simulink model "VTOLDynamics"  (R2026a)
settings: Solver=VariableStepAuto  StopTime=10
undefined symbols (not defined in the file): battery, contact, env, F, iniRoll, initPitch, iniYaw, Light, MIL, minPWM, motorPID, percWeightGain, tiltIni, uavParam, vIni, xGround, yGround, zGround
libraries: matrix_library x8, robotcorelib x4, aerolibasang x2, aerolibwind2 x2, aerolibobsolete x1, aerolibadyn x1, fl_lib x1, nesl_utility x1, sharedtransform x1
(part 1 of 2)
settings Model: DataDictionary=VTOLDynamicsData.sldd  Creator=The MathWorks, Inc.  LastModifiedBy=The MathWorks, Inc.
settings ModelReferenceCC: ModelReferenceNumInstancesAllowed=Single
settings GRTTargetCC: SubcomponentCodeInterfacePackaging=Nonreusable function
settings SimscapeCC: SimscapeNominalValues="[{\"value\":\"1\",\"unit\":\"A\"},{\"value\":\"1\",\"unit\":\"bar\"},{\"value\":\"1\",\"unit\":\"cm^2\"},{\"value\":\"1\",\"unit\":\"cm^3/s\"},{\"value\":\"1\",\"unit\":\"kJ/kg\"},{\"value\":\"1\",\"unit\":\"kW\"},{\"value\":\"1\",\"unit\":\"l\"},{\"value\":\"1\",\"unit\":\"N\"},{\"value\":\"1\",\"unit\":\"N*m\"},{\"value\":\"1\",\"unit\":\"V\"}]"  SimscapeLogType=none  SimscapeLogDataHistory=5000.0

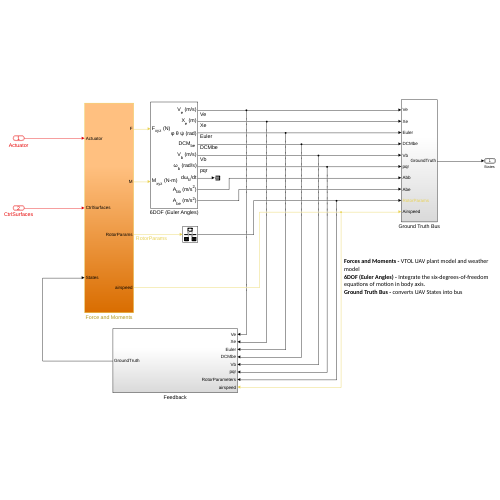
[thumbnail: Simulink's stored preview of the top-level diagram]
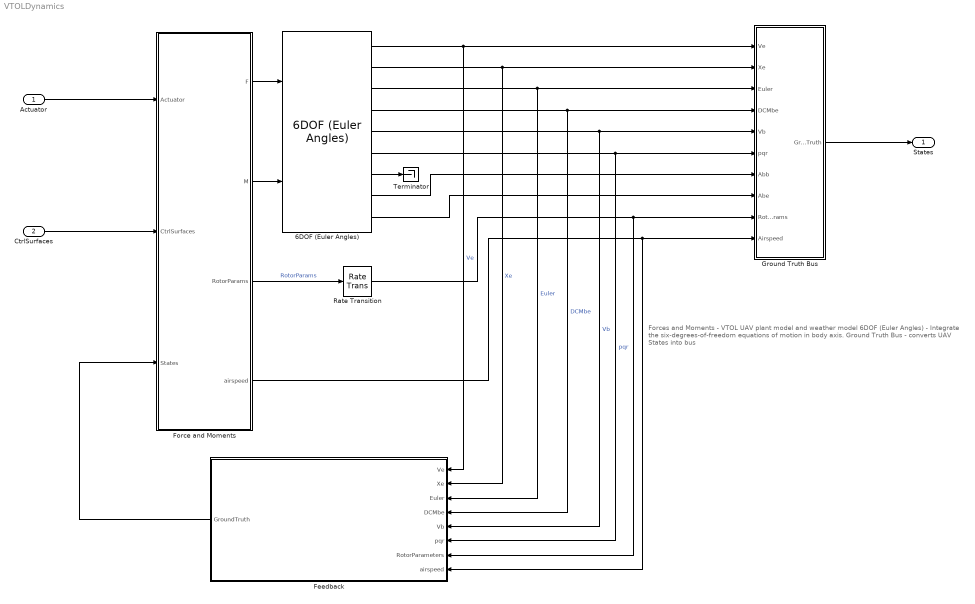
== system VTOLDynamics ==
  note: Forces and Moments - VTOL UAV plant model and weather model
      | 6DOF (Euler Angles) - Integrate the six-degrees-of-freedom equations of motion in body axis.
      | Ground Truth Bus - converts UAV States into bus
  Actuator : Inport  OutDataTypeStr=Bus: RotorCtrlBus  BusOutputAsStruct=on
  CtrlSurfaces : Inport  Port=2  OutDataTypeStr=Bus: FixedWingCtrlBus  BusOutputAsStruct=on
  6DOF (Euler Angles) : aerolibobsolete/6DOF (Euler Angles)  units=Metric (MKS)  mtype=Fixed  rep=Euler Angles  xme_0=[xGround, yGround, zGround]  Vm_0=[vIni 0 0]  eul_0=[iniRoll initPitch iniYaw]  pm_0=[0 0 0]  mass_0=6.031*percWeightGain  mass_e=0.5  mass_f=2.0  inertia=[uavParam.geom.Ixx 0 0; 0 uavParam.geom.Iyy 0; 0 0 uavParam.geom.Izz]  inertia_e=eye(3)  inertia_f=2*eye(3)  k_quat=1.0  vre_flag=on  abi_flag=on  aMode=0  xme_statename=''  Vm_statename=''  eul_statename=''  quat_statename=''  pm_statename=''  mass_statename=''
  Feedback : Subsystem
  Force and Moments : Subsystem
  Ground Truth Bus : Subsystem
  Rate Transition : RateTransition
  Terminator : Terminator
  "States " : Outport  OutDataTypeStr=Bus: stateBus  BusOutputAsStruct=on
  wires:
  6DOF (Euler Angles)/4 -> Feedback/4(DCMbe), Ground Truth Bus/4(DCMbe)  "DCMbe"
  Actuator/1 -> Force and Moments/1(Actuator)
  6DOF (Euler Angles)/2 -> Feedback/2(Xe), Ground Truth Bus/2(Xe)  "Xe"
  Force and Moments/4(airspeed) -> Ground Truth Bus/10(Airspeed), Feedback/8(airspeed)
  6DOF (Euler Angles)/1 -> Feedback/1(Ve), Ground Truth Bus/1(Ve)  "Ve"
  Force and Moments/3(RotorParams) -> Rate Transition/1  "RotorParams"
  6DOF (Euler Angles)/6 -> Feedback/6(pqr), Ground Truth Bus/6(pqr)  "pqr"
  CtrlSurfaces/1 -> Force and Moments/2(CtrlSurfaces)
  6DOF (Euler Angles)/7 -> Terminator/1
  6DOF (Euler Angles)/3 -> Feedback/3(Euler), Ground Truth Bus/3(Euler)  "Euler"
  6DOF (Euler Angles)/5 -> Feedback/5(Vb), Ground Truth Bus/5(Vb)  "Vb"
  Ground Truth Bus/1(GroundTruth) -> "States "/1
  6DOF (Euler Angles)/8 -> Ground Truth Bus/7(Abb)
  6DOF (Euler Angles)/9 -> Ground Truth Bus/8(Abe)
  Feedback/1(GroundTruth) -> Force and Moments/3(States)
  Force and Moments/1(F) -> 6DOF (Euler Angles)/1
  Force and Moments/2(M) -> 6DOF (Euler Angles)/2
  Rate Transition/1 -> Feedback/7(RotorParameters), Ground Truth Bus/9(RotorParams)

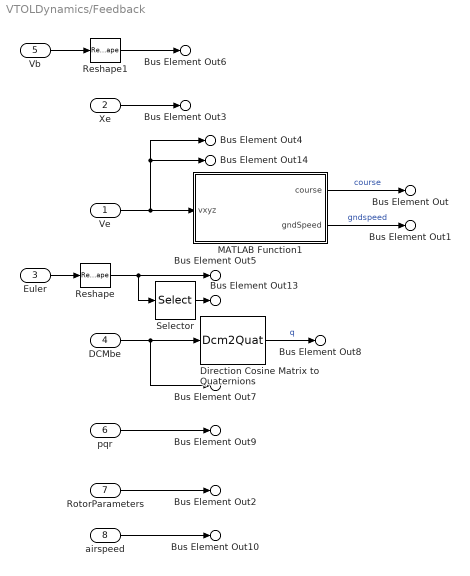
== system VTOLDynamics/Feedback ==
  Ve : Inport
  Xe : Inport  Port=2
  Euler : Inport  Port=3
  DCMbe : Inport  Port=4
  Vb : Inport  Port=5
  pqr : Inport  Port=6
  RotorParameters : Inport  Port=7
  airspeed : Inport  Port=8
  Direction Cosine Matrix to Quaternions : Dcm2Quat
  MATLAB Function1 : MATLAB Function  TreatAsAtomicUnit=on
  Reshape : Reshape  OutputDimensionality=Column vector (2-D)
  Reshape1 : Reshape  OutputDimensionality=Row vector (2-D)
  Selector : Selector  InputPortWidth=3  IndexOptions=Index vector (dialog)  Indices=[3 2 1]  OutputSizes=1
  Bus Element Out : Outport  PortName=GroundTruth  Element=course
  Bus Element Out1 : Outport  PortName=GroundTruth  Element=gndspeed
  Bus Element Out3 : Outport  PortName=GroundTruth  Element=Xe
  Bus Element Out4 : Outport  PortName=GroundTruth  Element=Ve
  Bus Element Out7 : Outport  PortName=GroundTruth  Element=DCMbe
  Bus Element Out8 : Outport  PortName=GroundTruth  Element=q
  Bus Element Out9 : Outport  PortName=GroundTruth  Element=pqr
  Bus Element Out6 : Outport  PortName=GroundTruth  Element=Vb
  Bus Element Out5 : Outport  PortName=GroundTruth  Element=Euler
  Bus Element Out13 : Outport  PortName=GroundTruth  Element=ypr
  Bus Element Out14 : Outport  PortName=GroundTruth  Element=Ve_ground
  Bus Element Out2 : Outport  PortName=GroundTruth  Element=RotorParameters
  Bus Element Out10 : Outport  PortName=GroundTruth  Element=airspeed
  wires:
  Reshape1/1 -> Bus Element Out6/1
  Reshape/1 -> Bus Element Out5/1, Selector/1
  Selector/1 -> Bus Element Out13/1
  pqr/1 -> Bus Element Out9/1
  Direction Cosine Matrix to Quaternions/1 -> Bus Element Out8/1  "q"
  Vb/1 -> Reshape1/1
  Euler/1 -> Reshape/1
  Xe/1 -> Bus Element Out3/1
  MATLAB Function1/2(gndSpeed) -> Bus Element Out1/1  "gndspeed"
  MATLAB Function1/1(course) -> Bus Element Out/1  "course"
  Ve/1 -> MATLAB Function1/1(vxyz), Bus Element Out4/1, Bus Element Out14/1
  DCMbe/1 -> Direction Cosine Matrix to Quaternions/1, Bus Element Out7/1
  RotorParameters/1 -> Bus Element Out2/1
  airspeed/1 -> Bus Element Out10/1

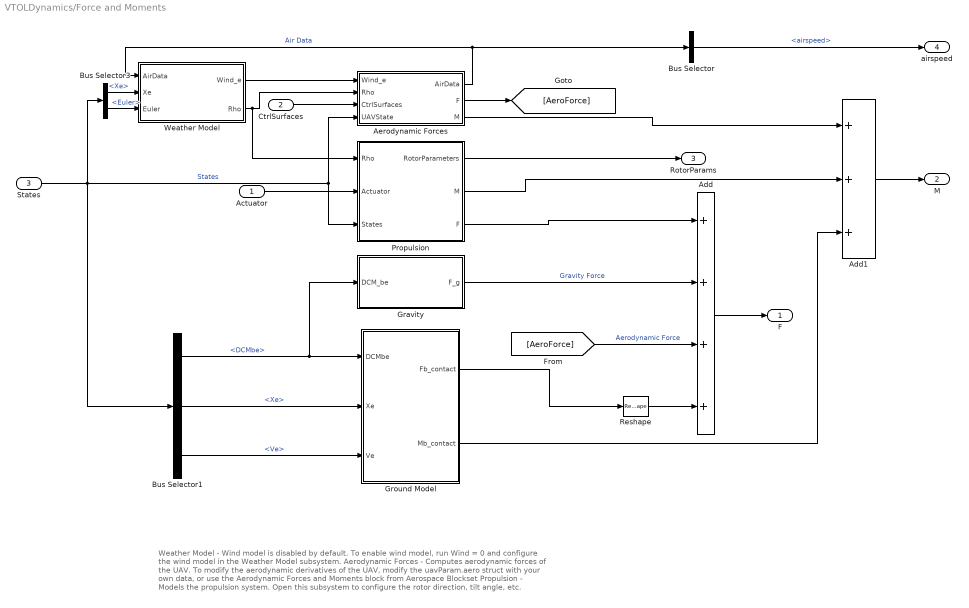
== system VTOLDynamics/Force and Moments ==
  note: Weather Model - Wind model is disabled by default. To enable wind model, run Wind = 0 and configure the wind model in the Weather Model subsystem.
      |
      | Aerodynamic Forces - Computes aerodynamic forces of the UAV. To modify the aerodynamic derivatives of the UAV, modify the uavParam.aero struct with your own data, or use the Aerodynamic Forces and Moments block from Aerospace Blockset
      |
      | Propulsion - Models the propulsion system. Open this subsystem to configure the rotor direction, tilt angle, etc.
  Actuator : Inport
  CtrlSurfaces : Inport  Port=2
  States : Inport  Port=3
  Add : Sum  Inputs=++++
  Add1 : Sum  Inputs=+++
  Aerodynamic Forces : Subsystem
  Bus Selector : BusSelector  OutputSignals=airspeed
  Bus Selector1 : BusSelector  OutputSignals=DCMbe,Xe,Ve
  Bus Selector3 : BusSelector  OutputSignals=Xe,Euler
  Gravity : Subsystem
  Ground Model : Subsystem  VariantControl=Groundon==1
  Propulsion : Subsystem  Variant=on
  Reshape : Reshape
  Weather Model : Subsystem  Variant=on  VariantControl=Weather Model
  F : Outport
  M : Outport  Port=2
  RotorParams : Outport  Port=3
  airspeed : Outport  Port=4
  wires:
  Gravity/1(F_g) -> Add/2  "Gravity Force"
  Add/1 -> F/1
  States/1 -> Bus Selector3/1, Bus Selector1/1, Propulsion/3(States), Aerodynamic Forces/4(UAVState)  "States"
  CtrlSurfaces/1 -> Aerodynamic Forces/3(CtrlSurfaces)
  Add1/1 -> M/1
  [AeroForce] -> Add/3  "Aerodynamic Force"
  Aerodynamic Forces/2(F) -> [AeroForce]
  Aerodynamic Forces/3(M) -> Add1/1
  Aerodynamic Forces/1(AirData) -> Weather Model/1(AirData), Bus Selector/1  "Air Data"
  Bus Selector3/1 -> Weather Model/2(Xe)  "<Xe>"
  Bus Selector3/2 -> Weather Model/3(Euler)  "<Euler>"
  Weather Model/1(Wind_e) -> Aerodynamic Forces/1(Wind_e)
  Weather Model/2(Rho) -> Aerodynamic Forces/2(Rho), Propulsion/1(Rho)
  Bus Selector1/3 -> Ground Model/3(Ve)  "<Ve>"
  Bus Selector1/2 -> Ground Model/2(Xe)  "<Xe>"
  Bus Selector1/1 -> Gravity/1(DCM_be), Ground Model/1(DCMbe)  "<DCMbe>"
  Ground Model/1(Fb_contact) -> Reshape/1
  Ground Model/2(Mb_contact) -> Add1/3
  Reshape/1 -> Add/4
  Bus Selector/1 -> airspeed/1  "<airspeed>"
  Actuator/1 -> Propulsion/2(Actuator)
  Propulsion/2(M) -> Add1/2
  Propulsion/3(F) -> Add/1
  Propulsion/1(RotorParameters) -> RotorParams/1

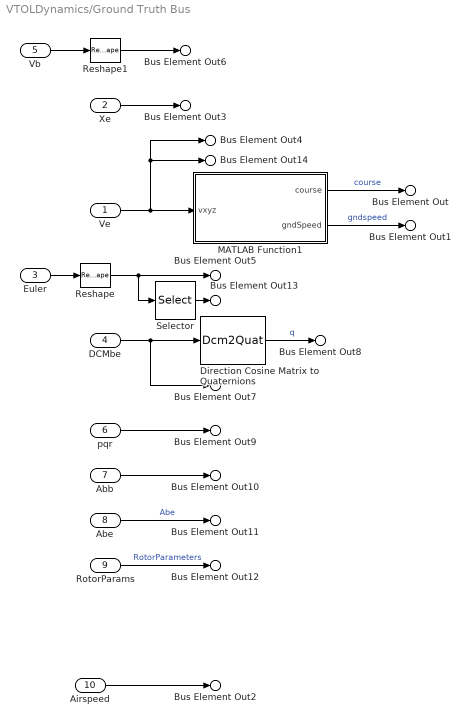
== system VTOLDynamics/Ground Truth Bus ==
  Ve : Inport
  Xe : Inport  Port=2
  Euler : Inport  Port=3
  DCMbe : Inport  Port=4
  Vb : Inport  Port=5
  pqr : Inport  Port=6
  Abb : Inport  Port=7
  Abe : Inport  Port=8
  RotorParams : Inport  Port=9
  Airspeed : Inport  Port=10
  Direction Cosine Matrix to Quaternions : Dcm2Quat
  MATLAB Function1 : MATLAB Function  TreatAsAtomicUnit=on
  Reshape : Reshape  OutputDimensionality=Column vector (2-D)
  Reshape1 : Reshape  OutputDimensionality=Row vector (2-D)
  Selector : Selector  InputPortWidth=3  IndexOptions=Index vector (dialog)  Indices=[3 2 1]  OutputSizes=1
  Bus Element Out : Outport  PortName=GroundTruth  Element=course
  Bus Element Out1 : Outport  PortName=GroundTruth  Element=gndspeed
  Bus Element Out2 : Outport  PortName=GroundTruth  Element=airspeed
  Bus Element Out3 : Outport  PortName=GroundTruth  Element=Xe
  Bus Element Out4 : Outport  PortName=GroundTruth  Element=Ve
  Bus Element Out7 : Outport  PortName=GroundTruth  Element=DCMbe
  Bus Element Out8 : Outport  PortName=GroundTruth  Element=q
  Bus Element Out9 : Outport  PortName=GroundTruth  Element=pqr
  Bus Element Out6 : Outport  PortName=GroundTruth  Element=Vb
  Bus Element Out10 : Outport  PortName=GroundTruth  Element=Abb
  Bus Element Out11 : Outport  PortName=GroundTruth  Element=Abe
  Bus Element Out5 : Outport  PortName=GroundTruth  Element=Euler
  Bus Element Out12 : Outport  PortName=GroundTruth  Element=RotorParameters
  Bus Element Out13 : Outport  PortName=GroundTruth  Element=ypr
  Bus Element Out14 : Outport  PortName=GroundTruth  Element=Ve_ground
  wires:
  DCMbe/1 -> Bus Element Out7/1, Direction Cosine Matrix to Quaternions/1
  Airspeed/1 -> Bus Element Out2/1
  Ve/1 -> Bus Element Out14/1, Bus Element Out4/1, MATLAB Function1/1(vxyz)
  MATLAB Function1/1(course) -> Bus Element Out/1  "course"
  MATLAB Function1/2(gndSpeed) -> Bus Element Out1/1  "gndspeed"
  Xe/1 -> Bus Element Out3/1
  Euler/1 -> Reshape/1
  Vb/1 -> Reshape1/1
  Direction Cosine Matrix to Quaternions/1 -> Bus Element Out8/1  "q"
  pqr/1 -> Bus Element Out9/1
  Abb/1 -> Bus Element Out10/1
  Abe/1 -> Bus Element Out11/1  "Abe"
  RotorParams/1 -> Bus Element Out12/1  "RotorParameters"
  Selector/1 -> Bus Element Out13/1
  Reshape/1 -> Selector/1, Bus Element Out5/1
  Reshape1/1 -> Bus Element Out6/1

== system VTOLDynamics/Force and Moments/Aerodynamic Forces ==
  Wind_e : Inport
  Rho : Inport  Port=2
  CtrlSurfaces : Inport  Port=3
  UAVState : Inport  Port=4
  Bus Selector2 : BusSelector  OutputSignals=DCMbe,Ve,pqr
  Compute Air Data : Subsystem  TreatAsAtomicUnit=on  VariantControl=use_aerospace_blocks == 1
  Compute Body Frame Forces and Moments : Subsystem
  Matrix Multiply : Product  Multiplication=Matrix(*)
  Vair : Sum  Inputs=+-  InputSameDT=on  SaturateOnIntegerOverflow=on  OutDataTypeStr=Inherit: Same as first input
  AirData : Outport  VectorParamsAs1DForOutWhenUnconnected=off
  F : Outport  Port=2
  M : Outport  Port=3
  wires:
  Bus Selector2/2 -> Vair/1  "<Ve>"
  UAVState/1 -> Bus Selector2/1
  Compute Body Frame Forces and Moments/1(F_b) -> F/1
  CtrlSurfaces/1 -> Compute Body Frame Forces and Moments/2(CtrlSurfaces)
  Compute Air Data/1(AirData) -> Compute Body Frame Forces and Moments/1(AirData), AirData/1
  Bus Selector2/3 -> Compute Body Frame Forces and Moments/4(p,q,r)  "<pqr>"
  Compute Body Frame Forces and Moments/2(M_b) -> M/1
  Matrix Multiply/1 -> Compute Body Frame Forces and Moments/3(Vb), Compute Air Data/1(Vb)
  Rho/1 -> Compute Air Data/2(Rho)
  Vair/1 -> Matrix Multiply/2
  Bus Selector2/1 -> Matrix Multiply/1  "<DCMbe>"
  Wind_e/1 -> Vair/2

== system VTOLDynamics/Force and Moments/Gravity ==
  DCM_be : Inport
  Constant : Constant  Value=[0 0 uavParam.aero.g]'
  Gain : Gain  Gain=uavParam.geom.mass*percWeightGain
  Matrix Multiply : Product  Multiplication=Matrix(*)
  F_g : Outport
  wires:
  Matrix Multiply/1 -> Gain/1
  Constant/1 -> Matrix Multiply/2
  DCM_be/1 -> Matrix Multiply/1
  Gain/1 -> F_g/1

== system VTOLDynamics/Force and Moments/Ground Model ==
  note: Body is assumed to be a rigid point mass on ground for contact force calculations.
      |
      | Normal force is modelled as a spring mass damper.
      |
      | Friction is modelled using Soft Coulomb model.
  DCMbe : Inport
  Xe : Inport  Port=2
  Ve : Inport  Port=3
  Constant : Constant  Value=[0 0 0]  SampleTime=-1
  Friction Force : Subsystem
  Matrix Multiply : Product  Multiplication=Matrix(*)
  Mux1 : Mux  Inputs=2
  Normal Force : Subsystem
  Selector : Selector  InputPortWidth=3  IndexOptions=Index vector (dialog)  Indices=[3]  OutputSizes=1
  Selector1 : Selector  InputPortWidth=3  IndexOptions=Index vector (dialog)  Indices=[3]  OutputSizes=1
  Selector2 : Selector  InputPortWidth=3  IndexOptions=Index vector (dialog)  Indices=[1,2]  OutputSizes=1
  Unary Minus1 : UnaryMinus
  Fb_contact : Outport
  Mb_contact : Outport  Port=2
  wires:
  Xe/1 -> Selector/1
  Ve/1 -> Selector2/1, Selector1/1
  Selector1/1 -> Normal Force/1(Vz)
  Selector/1 -> Normal Force/2(Z)
  DCMbe/1 -> Matrix Multiply/1
  Matrix Multiply/1 -> Fb_contact/1
  Normal Force/1(Normal) -> Friction Force/2(Fn), Unary Minus1/1
  Mux1/1 -> Matrix Multiply/2
  Unary Minus1/1 -> Mux1/2
  Selector2/1 -> Friction Force/1(V)
  Friction Force/1(Friction) -> Mux1/1
  Constant/1 -> Mb_contact/1

== system VTOLDynamics/Force and Moments/Propulsion ==
  note: 1) Add Subsystem or Model blocks as valid variant choices.
      | 2) You cannot connect blocks at this level. At simulation, connectivity is automatically
      | determined, based on the active variant and port name matching.
  Rho : Inport
  Actuator : Inport  Port=2
  States : Inport  Port=3
  Electric Propulsion : Subsystem  VariantControl=ElectricPropulsion == 1
  Propulsion : Subsystem  VariantControl=ElectricPropulsion == 0
  RotorParameters : Outport
  M : Outport  Port=2
  F : Outport  Port=3

== system VTOLDynamics/Force and Moments/Weather Model ==
  AirData : Inport
  Xe : Inport  Port=2
  Euler : Inport  Port=3
  Simple Model : Subsystem  VariantControl=Wind==0
  Weather Model : Subsystem  VariantControl=Wind==1
  Wind_e : Outport
  Rho : Outport  Port=2

== system VTOLDynamics/Force and Moments/Aerodynamic Forces/Compute Air Data ==
  Vb : Inport  PortDimensions=3
  Rho : Inport  Port=2
  Bus Creator : BusCreator  Inputs=4
  Constant : Constant  Value=5/57.296
  Dynamic Pressure : aerolibasang/Dynamic Pressure
  "Incidence, Sideslip, & Airspeed" : aerolibasang/Incidence, Sideslip, & Airspeed
  Saturation : Saturate  UpperLimit=14*pi/180  LowerLimit=-14*pi/180
  Sum : Sum  Inputs=|++
  To Workspace : ToWorkspace  VariableName=Alpha  SaveFormat=Timeseries  SampleTime=-1
  AirData : Outport  VectorParamsAs1DForOutWhenUnconnected=off
  wires:
  Bus Creator/1 -> AirData/1
  "Incidence, Sideslip, & Airspeed"/1 -> Sum/2, Bus Creator/1  "alpha"
  Rho/1 -> Dynamic Pressure/2
  "Incidence, Sideslip, & Airspeed"/3 -> Bus Creator/3  "airspeed"
  Dynamic Pressure/1 -> Bus Creator/4  "q"
  Vb/1 -> "Incidence, Sideslip, & Airspeed"/1, Dynamic Pressure/1
  "Incidence, Sideslip, & Airspeed"/2 -> Saturation/1  "beta"
  Saturation/1 -> Bus Creator/2  "beta"
  Constant/1 -> Sum/1
  Sum/1 -> To Workspace/1

== system VTOLDynamics/Force and Moments/Aerodynamic Forces/Compute Body Frame Forces and Moments ==
  AirData : Inport
  CtrlSurfaces : Inport  Port=2
  Vb : Inport  Port=3
  p,q,r : Inport  Port=4
  "Aerodynamic Forces and Moments " : aerolibadyn/Aerodynamic Forces and Moments   inputAxes=Wind  outputForceAxes=Body  outputMomentAxes=Body  S=uavParam.geom.b*uavParam.geom.c  b=uavParam.geom.b  cbar=uavParam.geom.c
  Constant1 : Constant  Value=[0 0 0]
  Constant2 : Constant  Value=[0 0 0]
  Wind frame F& M : Subsystem
  F_b : Outport  Unit=kg*m/s^2  VectorParamsAs1DForOutWhenUnconnected=off
  M_b : Outport  Port=2  Unit=kg*m/s  VectorParamsAs1DForOutWhenUnconnected=off
  wires:
  p,q,r/1 -> Wind frame F& M/3(p,q,r)
  "Aerodynamic Forces and Moments "/2 -> M_b/1
  "Aerodynamic Forces and Moments "/1 -> F_b/1
  CtrlSurfaces/1 -> Wind frame F& M/2(CtrlSurfaces)
  AirData/1 -> Wind frame F& M/1(Airdata)
  Vb/1 -> "Aerodynamic Forces and Moments "/5
  Constant1/1 -> "Aerodynamic Forces and Moments "/3
  Constant2/1 -> "Aerodynamic Forces and Moments "/4
  Wind frame F& M/1(coef) -> "Aerodynamic Forces and Moments "/1  "FM_W"
  Wind frame F& M/2(q) -> "Aerodynamic Forces and Moments "/2

== system VTOLDynamics/Force and Moments/Ground Model/Friction Force ==
  V : Inport
  Fn : Inport  Port=2
  Product : Product
  Soft Coulomb Friction : Subsystem
  Unary Minus : UnaryMinus
  Friction : Outport
  wires:
  Unary Minus/1 -> Friction/1
  Fn/1 -> Product/2
  Soft Coulomb Friction/1(Out1) -> Product/1
  Product/1 -> Unary Minus/1
  V/1 -> Soft Coulomb Friction/1(V)

== system VTOLDynamics/Force and Moments/Ground Model/Normal Force ==
  Vz : Inport
  Z : Inport  Port=2
  Add : Sum
  Constant : Constant  Value=0  SampleTime=-1
  Damper : Gain  Gain=-sqrt(contact.spring*uavParam.geom.mass)
  Saturation : Saturate  UpperLimit=inf  LowerLimit=0  ZeroCross=off
  Spring Kp : Gain  Gain=-contact.spring
  Switch : Switch  Criteria=u2 > Threshold  SaturateOnIntegerOverflow=off  InputSameDT=off
  Unary Minus : UnaryMinus
  Unary Minus1 : UnaryMinus
  Normal : Outport
  wires:
  Add/1 -> Switch/3
  Constant/1 -> Switch/1
  Z/1 -> Unary Minus/1
  Switch/1 -> Saturation/1
  Damper/1 -> Add/2
  Spring Kp/1 -> Add/1
  Vz/1 -> Unary Minus1/1
  Saturation/1 -> Normal/1
  Unary Minus/1 -> Spring Kp/1, Switch/2
  Unary Minus1/1 -> Damper/1

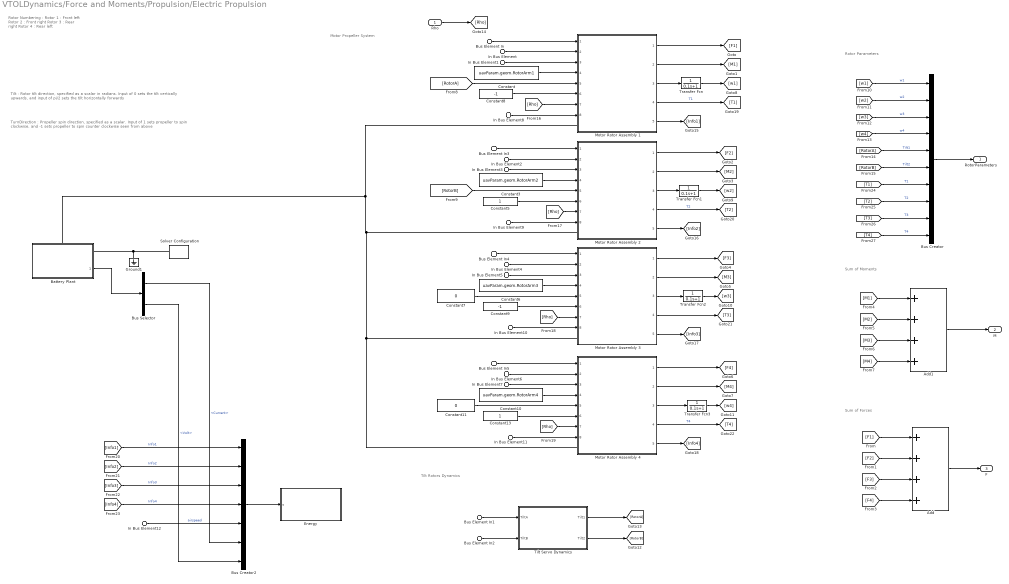
== system VTOLDynamics/Force and Moments/Propulsion/Electric Propulsion ==
  note: Rotor Parameters
  note: Sum of Forces
  note: Sum of Moments
  note: Tilt Rotors Dynamics
  note: Rotor Numbering :
      | Rotor 1 : Front left
      | Rotor 2 : Front right
      | Rotor 3 : Rear right
      | Rotor 4 : Rear left
  note: Tilt : Rotor tilt direction, specified as a scalar in radians. Input of 0 sets the tilt vertically upwards, and input of pi/2 sets the tilt horizontally forwards
  note: TurnDirection : Propeller spin direction, specified as a scalar. Input of 1 sets propeller to spin clockwise, and -1 sets propeller to spin counter clockwise seen from above
  note: Motor Propeller
      | System
  Rho : Inport
  Bus Element In : Inport  Port=2  PortName=Actuator  Element=w1
  Bus Element In1 : Inport  Port=2  PortName=Actuator  Element=Tilt1
  Bus Element In2 : Inport  Port=2  PortName=Actuator  Element=Tilt2
  Bus Element In3 : Inport  Port=2  PortName=Actuator  Element=w2
  Bus Element In5 : Inport  Port=2  PortName=Actuator  Element=w4
  Bus Element In4 : Inport  Port=2  PortName=Actuator  Element=w3
  In Bus Element{,2,4,6} (4 alike) : Inport  Port=3  PortName=States  Element=Vb
  In Bus Element{1,3,5,7} (4 alike) : Inport  Port=3  PortName=States  Element=pqr
  In Bus Element8 : Inport  Port=3  PortName=States  Element=RotorParameters.T1
  In Bus Element9 : Inport  Port=3  PortName=States  Element=RotorParameters.T2
  In Bus Element10 : Inport  Port=3  PortName=States  Element=RotorParameters.T3
  In Bus Element11 : Inport  Port=3  PortName=States  Element=RotorParameters.T4
  In Bus Element12 : Inport  Port=3  PortName=States  Element=airspeed
  Add : Sum  Inputs=++++
  Add1 : Sum  Inputs=++++
  Battery Plant : Subsystem  ReferencedSubsystem=BatteryPlantModel_Simple
      settings: PortSchema="{\"entries\":[{\"content\":{\"sides\":[{\"content\":{},\"type\":\"ConnectorPlacement.EquallySpacedRectSide\",\"uuid\":\"ba36f307-b33b-4535-ba0b-2e0bfd99fc4d\"},{\"content\":{\"connectorIds\":[\"RConn2\",\"Out1\"],\"side\":\"RIGHT\"},\"type\":\"ConnectorPlacement.EquallySpacedRectSide\",\"uuid\":\"89704593-04c2-4c1a-a3b9-13b3f56a74b5\"},{\"content\":{\"connectorIds\":[\"RConn1\"],\"side\":\"TOP\"},\"type\":\"ConnectorPlacement.EquallySpacedRectSide\",\"uuid\":\"1daeac74-7d2b-4aa4-8837-06dc1649b516\"},{\"content\":{\"side\":\"BOTTOM\"},\"type\":\"ConnectorPlacement.EquallySpacedRectSide\",\"uuid\":\"a55355a8-f534-49c8-a897-d3f7ff506222\"}]},\"type\":\"ConnectorPlacement.EquallySpacedConnector\",\"uuid\":\"2c693ef8-3b08-48d7-935c-b55223a280fc\"}],\"packageUris\":[\"http://schema.mathworks.com/mf0/Connector/R2020b\"],\"version\":\"1.0\"}"
  Bus Creator : BusCreator  Inputs=10  OutDataTypeStr=Bus: RotorCtrlBus
  Bus Creator2 : BusCreator  Inputs=7
  Bus Selector : BusSelector  OutputSignals=Current,Volt
  Constant : Constant  Value=uavParam.geom.RotorArm1
  Constant10 : Constant  Value=uavParam.geom.RotorArm4
  Constant11 : Constant  Value=0
  Constant13 : Constant
  Constant3 : Constant  Value=uavParam.geom.RotorArm2
  Constant5 : Constant
  Constant6 : Constant  Value=uavParam.geom.RotorArm3
  Constant7 : Constant  Value=0
  Constant8 : Constant  Value=-1
  Constant9 : Constant  Value=-1
  Energy : Subsystem
      mask Display:
      | %disp(get_param(gcb, 'Name'))
      | disp(['{\bf\fontsize{12}' get_param(gcb, 'Name') '}'], 'texmode','on');
  Ground1 : fl_lib/Electrical/Electrical Elements/Electrical Reference
  Motor Rotor Assembly {1..4} (4 alike) : Subsystem  ReferencedSubsystem=MotorPropellerSystem  Kp=motorPID.Kpp  Ki=motorPID.Kii  Kd=motorPID.Kdd  N=motorPID.N
  Solver Configuration : nesl_utility/Solver Configuration  PhysicalDomain=network_engine_domain  SubClassName=solver  LeftPortType=input  RightPortType=generic  Tones=[]  Harmonics=[]  SimulateNoise=off  Profile=off  UseLocalSampling=off  EnableSwitchedLinearOptims=on  FrequencyDomain=off  UseCCode=off  RelTol=0.001  AbsTol=0.001  MinStep=1e-09  ToWorkspace=off  RevertToSquareIcSolve=off  NumHomotopyIterations=100  PhasorMode=off  PhasorModeNumHarmonics=1  ConsistencySolver=NEWTON_XTOL_AFTER_FTOL  CanonicalOrdering=UNORDERED  OptimizeIntermediates=UNOPTIMIZED  IndexReductionMethod=DerivativeReplacement  DoDC=off  ResidualTolerance=1e-09  ConsistencyTolSource=GLOBAL  ConsistencyAbsTol=0.001  ConsistencyRelTol=0.001  ConsistencyTolFactor=0.001  UseLocalSolver=on  LocalSolverChoice=NE_BACKWARD_EULER_ADVANCER  ResolveIndetEquations=on  FunctionEvalNumThread=1  LocalSolverSampleTime=0.01  DoFixedCost=off  MaxNonlinIter=3  MaxModeIter=2  ComputeImpulses=off  ImpulseIterations=2  LinearAlgebra=auto  LinearAlgebraNumThread=0  EquationFormulation=NE_TIME_EF  DelaysMemoryBudget=1024  AutomaticFiltering=on  FilteringTimeConstant=0.001  PartitionStorageMethod=AS_NEEDED  PartitionMemoryBudget=1024  PartitionMethod=ROBUST  MultibodyUseLocalSolver=off  MultibodyLocalSolverChoice=ODE1  MultibodyLocalSolverSampleTime=0.001
  Tilt Servo Dynamics : Subsystem
  Transfer Fcn{,1..3} (4 alike) : TransferFcn  Denominator=[0.1 1]
  RotorParameters : Outport
  M : Outport  Port=2
  F : Outport  Port=3
  wires:
  [Rho] -> Motor Rotor Assembly 4/7
  [Rho] -> Motor Rotor Assembly 2/7
  [RotorB] -> Motor Rotor Assembly 2/5
  [Rho] -> Motor Rotor Assembly 1/7
  Rho/1 -> [Rho]
  Transfer Fcn3/1 -> [w4]
  Transfer Fcn2/1 -> [w3]
  Transfer Fcn1/1 -> [w2]
  Transfer Fcn/1 -> [w1]
  Bus Element In2/1 -> Tilt Servo Dynamics/2(TiltB)
  Bus Element In1/1 -> Tilt Servo Dynamics/1(TiltA)
  Tilt Servo Dynamics/2(Tilt2) -> [RotorB]
  Tilt Servo Dynamics/1(Tilt1) -> [RotorA]
  Bus Element In5/1 -> Motor Rotor Assembly 4/1
  Bus Element In3/1 -> Motor Rotor Assembly 2/1
  Bus Element In/1 -> Motor Rotor Assembly 1/1
  [RotorB] -> Bus Creator/6  "Tilt2"
  [RotorA] -> Bus Creator/5  "Tilt1"
  Bus Creator/1 -> RotorParameters/1
  [w4] -> Bus Creator/4  "w4"
  [w3] -> Bus Creator/3  "w3"
  [w2] -> Bus Creator/2  "w2"
  [w1] -> Bus Creator/1  "w1"
  Motor Rotor Assembly 4/3 -> Transfer Fcn3/1
  Motor Rotor Assembly 2/3 -> Transfer Fcn1/1
  Motor Rotor Assembly 1/3 -> Transfer Fcn/1
  [M1] -> Add1/1
  [M2] -> Add1/2
  [M3] -> Add1/3
  Add1/1 -> M/1
  [M4] -> Add1/4
  [F4] -> Add/4
  [F3] -> Add/3
  [F2] -> Add/2
  [F1] -> Add/1
  Motor Rotor Assembly 4/2 -> [M4]
  In Bus Element7/1 -> Motor Rotor Assembly 4/3
  Constant11/1 -> Motor Rotor Assembly 4/5
  Constant13/1 -> Motor Rotor Assembly 4/6
  Constant10/1 -> Motor Rotor Assembly 4/4
  In Bus Element6/1 -> Motor Rotor Assembly 4/2
  Motor Rotor Assembly 4/1 -> [F4]
  Motor Rotor Assembly 2/2 -> [M2]
  In Bus Element3/1 -> Motor Rotor Assembly 2/3
  Constant5/1 -> Motor Rotor Assembly 2/6
  Constant3/1 -> Motor Rotor Assembly 2/4
  In Bus Element2/1 -> Motor Rotor Assembly 2/2
  Motor Rotor Assembly 2/1 -> [F2]
  Motor Rotor Assembly 1/2 -> [M1]
  Motor Rotor Assembly 1/1 -> [F1]
  Constant8/1 -> Motor Rotor Assembly 1/6
  Add/1 -> F/1
  [RotorA] -> Motor Rotor Assembly 1/5
  Constant/1 -> Motor Rotor Assembly 1/4
  In Bus Element1/1 -> Motor Rotor Assembly 1/3
  In Bus Element/1 -> Motor Rotor Assembly 1/2
  Battery Plant/1 -> Bus Selector/1
  In Bus Element9/1 -> Motor Rotor Assembly 2/8
  In Bus Element8/1 -> Motor Rotor Assembly 1/8
  In Bus Element11/1 -> Motor Rotor Assembly 4/8
  Motor Rotor Assembly 1/5 -> [Info1]
  Motor Rotor Assembly 2/5 -> [Info2]
  Motor Rotor Assembly 4/5 -> [Info4]
  [Info1] -> Bus Creator2/1  "Info1"
  [Info2] -> Bus Creator2/2  "Info2"
  [Info3] -> Bus Creator2/3  "Info3"
  [Info4] -> Bus Creator2/4  "Info4"
  In Bus Element12/1 -> Bus Creator2/5  "airspeed"
  Bus Selector/1 -> Bus Creator2/6  "<Current>"
  Bus Selector/2 -> Bus Creator2/7  "<Volt>"
  Bus Creator2/1 -> Energy/1(s)
  Motor Rotor Assembly 1/4 -> [T1]  "T1"
  Motor Rotor Assembly 2/4 -> [T2]  "T2"
  Motor Rotor Assembly 4/4 -> [T4]  "T4"
  [T1] -> Bus Creator/7  "T1"
  [T2] -> Bus Creator/8  "T2"
  [T3] -> Bus Creator/9  "T3"
  [T4] -> Bus Creator/10  "T4"
  Bus Element In4/1 -> Motor Rotor Assembly 3/1
  In Bus Element4/1 -> Motor Rotor Assembly 3/2
  In Bus Element5/1 -> Motor Rotor Assembly 3/3
  Constant6/1 -> Motor Rotor Assembly 3/4
  Constant7/1 -> Motor Rotor Assembly 3/5
  Constant9/1 -> Motor Rotor Assembly 3/6
  [Rho] -> Motor Rotor Assembly 3/7
  In Bus Element10/1 -> Motor Rotor Assembly 3/8
  Motor Rotor Assembly 3/5 -> [Info3]
  Motor Rotor Assembly 3/4 -> [T3]
  Motor Rotor Assembly 3/3 -> Transfer Fcn2/1
  Motor Rotor Assembly 3/2 -> [M3]
  Motor Rotor Assembly 3/1 -> [F3]
  connections:
  Solver Configuration/RConn1 -- Ground1/LConn1 -- Battery Plant/RConn2
  Motor Rotor Assembly 1/LConn1 -- Battery Plant/RConn1 -- Motor Rotor Assembly 2/LConn1 -- Motor Rotor Assembly 4/LConn1 -- Motor Rotor Assembly 3/LConn1

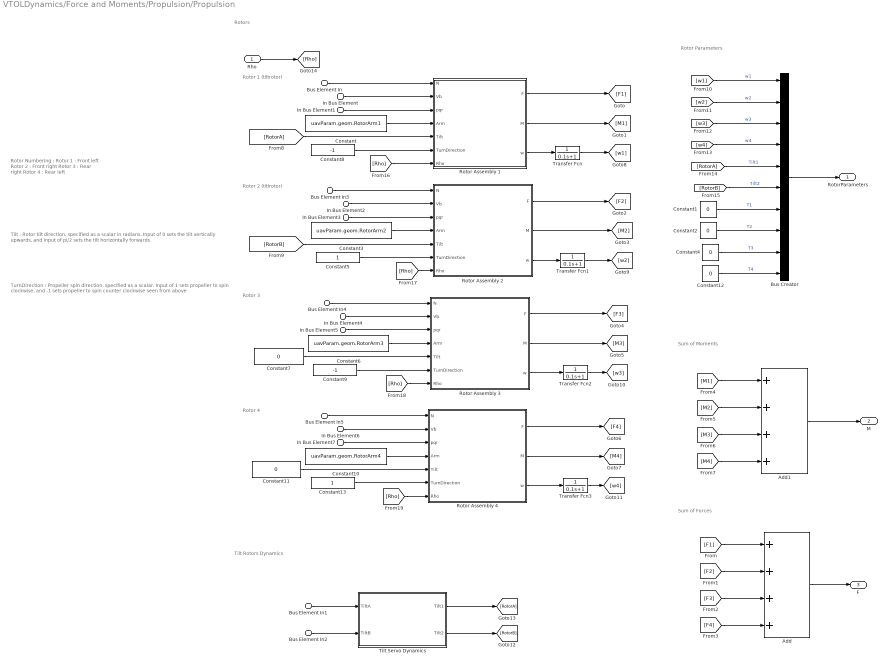
== system VTOLDynamics/Force and Moments/Propulsion/Propulsion ==
  note: TurnDirection : Propeller spin direction, specified as a scalar. Input of 1 sets propeller to spin clockwise, and -1 sets propeller to spin counter clockwise seen from above
  note: Tilt : Rotor tilt direction, specified as a scalar in radians. Input of 0 sets the tilt vertically upwards, and input of pi/2 sets the tilt horizontally forwards
  note: Rotor Numbering :
      | Rotor 1 : Front left
      | Rotor 2 : Front right
      | Rotor 3 : Rear right
      | Rotor 4 : Rear left
  note: Tilt Rotors Dynamics
  note: Sum of Moments
  note: Rotor 1
      | (tiltrotor)
  note: Rotors
  note: Rotor 2
      | (titlrotor)
  note: Rotor 3
  note: Rotor 4
  note: Sum of Forces
  note: Rotor Parameters
  Rho : Inport
  Bus Element In : Inport  Port=2  PortName=Actuator  Element=w1
  Bus Element In1 : Inport  Port=2  PortName=Actuator  Element=Tilt1
  Bus Element In2 : Inport  Port=2  PortName=Actuator  Element=Tilt2
  Bus Element In3 : Inport  Port=2  PortName=Actuator  Element=w2
  Bus Element In5 : Inport  Port=2  PortName=Actuator  Element=w4
  Bus Element In4 : Inport  Port=2  PortName=Actuator  Element=w3
  In Bus Element{,2,4,6} (4 alike) : Inport  Port=3  PortName=States  Element=Vb
  In Bus Element{1,3,5,7} (4 alike) : Inport  Port=3  PortName=States  Element=pqr
  Add : Sum  Inputs=++++
  Add1 : Sum  Inputs=++++
  Bus Creator : BusCreator  Inputs=10  OutDataTypeStr=Bus: RotorCtrlBus
  Constant : Constant  Value=uavParam.geom.RotorArm1
  Constant{1..2,4,7,11..12} (6 alike) : Constant  Value=0
  Constant10 : Constant  Value=uavParam.geom.RotorArm4
  Constant13 : Constant
  Constant3 : Constant  Value=uavParam.geom.RotorArm2
  Constant5 : Constant
  Constant6 : Constant  Value=uavParam.geom.RotorArm3
  Constant8 : Constant  Value=-1
  Constant9 : Constant  Value=-1
  Rotor Assembly 1 : Subsystem
  Rotor Assembly 2 : Subsystem
  "Rotor Assembly 3 " : Subsystem
  Rotor Assembly 4 : Subsystem
  Tilt Servo Dynamics : Subsystem
  Transfer Fcn{,1..3} (4 alike) : TransferFcn  Denominator=[0.1 1]
  RotorParameters : Outport
  M : Outport  Port=2
  F : Outport  Port=3
  wires:
  In Bus Element/1 -> Rotor Assembly 1/2(Vb)
  In Bus Element1/1 -> Rotor Assembly 1/3(pqr)
  Constant/1 -> Rotor Assembly 1/4(Arm)
  [RotorA] -> Rotor Assembly 1/5(Tilt)
  Add/1 -> F/1
  Constant8/1 -> Rotor Assembly 1/6(TurnDirection)
  Rotor Assembly 1/1(F) -> [F1]
  Rotor Assembly 1/2(M) -> [M1]
  Rotor Assembly 2/1(F) -> [F2]
  In Bus Element2/1 -> Rotor Assembly 2/2(Vb)
  Constant3/1 -> Rotor Assembly 2/4(Arm)
  Constant5/1 -> Rotor Assembly 2/6(TurnDirection)
  In Bus Element3/1 -> Rotor Assembly 2/3(pqr)
  Rotor Assembly 2/2(M) -> [M2]
  "Rotor Assembly 3 "/1(F) -> [F3]
  In Bus Element4/1 -> "Rotor Assembly 3 "/2(Vb)
  Constant6/1 -> "Rotor Assembly 3 "/4(Arm)
  Constant9/1 -> "Rotor Assembly 3 "/6(TurnDirection)
  Constant7/1 -> "Rotor Assembly 3 "/5(Tilt)
  In Bus Element5/1 -> "Rotor Assembly 3 "/3(pqr)
  "Rotor Assembly 3 "/2(M) -> [M3]
  Rotor Assembly 4/1(F) -> [F4]
  In Bus Element6/1 -> Rotor Assembly 4/2(Vb)
  Constant10/1 -> Rotor Assembly 4/4(Arm)
  Constant13/1 -> Rotor Assembly 4/6(TurnDirection)
  Constant11/1 -> Rotor Assembly 4/5(Tilt)
  In Bus Element7/1 -> Rotor Assembly 4/3(pqr)
  Rotor Assembly 4/2(M) -> [M4]
  [F1] -> Add/1
  [F2] -> Add/2
  [F3] -> Add/3
  [F4] -> Add/4
  [M4] -> Add1/4
  Add1/1 -> M/1
  [M3] -> Add1/3
  [M2] -> Add1/2
  [M1] -> Add1/1
  Rotor Assembly 1/3(w) -> Transfer Fcn/1
  Rotor Assembly 2/3(w) -> Transfer Fcn1/1
  "Rotor Assembly 3 "/3(w) -> Transfer Fcn2/1
  Rotor Assembly 4/3(w) -> Transfer Fcn3/1
  Bus Element In/1 -> Rotor Assembly 1/1(N)
  Bus Element In3/1 -> Rotor Assembly 2/1(N)
  Bus Element In4/1 -> "Rotor Assembly 3 "/1(N)
  Bus Element In5/1 -> Rotor Assembly 4/1(N)
  Tilt Servo Dynamics/1(Tilt1) -> [RotorA]
  Tilt Servo Dynamics/2(Tilt2) -> [RotorB]
  Bus Element In1/1 -> Tilt Servo Dynamics/1(TiltA)
  Bus Element In2/1 -> Tilt Servo Dynamics/2(TiltB)
  Transfer Fcn/1 -> [w1]
  Transfer Fcn1/1 -> [w2]
  Transfer Fcn2/1 -> [w3]
  Transfer Fcn3/1 -> [w4]
  Rho/1 -> [Rho]
  [Rho] -> Rotor Assembly 1/7(Rho)
  [RotorB] -> Rotor Assembly 2/5(Tilt)
  [Rho] -> Rotor Assembly 2/7(Rho)
  [Rho] -> "Rotor Assembly 3 "/7(Rho)
  [Rho] -> Rotor Assembly 4/7(Rho)
  [w1] -> Bus Creator/1  "w1"
  [w4] -> Bus Creator/4  "w4"
  [RotorB] -> Bus Creator/6  "Tilt2"
  [RotorA] -> Bus Creator/5  "Tilt1"
  Bus Creator/1 -> RotorParameters/1
  [w2] -> Bus Creator/2  "w2"
  [w3] -> Bus Creator/3  "w3"
  Constant1/1 -> Bus Creator/7  "T1"
  Constant2/1 -> Bus Creator/8  "T2"
  Constant4/1 -> Bus Creator/9  "T3"
  Constant12/1 -> Bus Creator/10  "T4"

== system VTOLDynamics/Force and Moments/Weather Model/Simple Model ==
  AirData : Inport
  Xe : Inport  Port=2
  Euler : Inport  Port=3
  Constant : Constant  Value=[ 0 0 0]
      settings: AttributesFormatString=%<Value>
  Constant1 : Constant  Value=uavParam.aero.rho
  Terminator : Terminator
  Terminator1 : Terminator
  Terminator3 : Terminator
  Wind_e : Outport  Unit=m/s  VectorParamsAs1DForOutWhenUnconnected=off
  " Rho" : Outport  Port=2  VectorParamsAs1DForOutWhenUnconnected=off
  wires:
  AirData/1 -> Terminator/1
  Constant/1 -> Wind_e/1
  Euler/1 -> Terminator1/1
  Xe/1 -> Terminator3/1
  Constant1/1 -> " Rho"/1

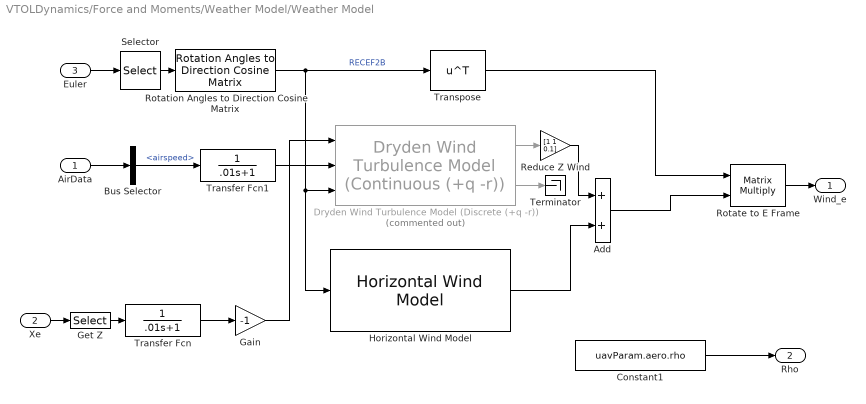
== system VTOLDynamics/Force and Moments/Weather Model/Weather Model ==
  AirData : Inport
  Xe : Inport  Port=2
  Euler : Inport  Port=3
  Add : Sum  Inputs=2
  Bus Selector : BusSelector  OutputSignals=airspeed
  Constant1 : Constant  Value=uavParam.aero.rho
  Dryden Wind Turbulence Model (Discrete (+q -r)) : aerolibwind2/Dryden Wind Turbulence Model  (Continuous (+q -r))  Commented=on  units=Metric (MKS)  spec=MIL-F-8785C  model=Discrete Dryden (+q -r)  W20=env.windBase/4  Wdeg=env.windDirTurb  TurbProb=10^-2 - Light  L_high=533.4  Wingspan=uavParam.geom.b  ts=0.005  Seed=[23341 23342 23343 23344]  T_on=on
  Gain : Gain  Gain=-1
      settings: AttributesFormatString=Z to Alt
  Get Z : Selector  InputPortWidth=3  IndexOptions=Index vector (dialog)  Indices=[3]  OutputSizes=[(-2)]
  Horizontal Wind Model : aerolibwind2/Horizontal Wind Model  units=Metric (MKS)  Vw_source=Internal  Vwind=8  W_source=Internal  Wdeg=env.windDirHor
  Reduce Z Wind : Gain  Gain=[1 1 0.1]
      settings: AttributesFormatString=%<Gain>
  Rotate to E Frame : Product  Multiplication=Matrix(*)
  Rotation Angles to Direction Cosine Matrix : sharedtransform/Rotation Angles to Direction Cosine Matrix  rotationOrder=ZYX  aMode=aMode
  Selector : Selector  InputPortWidth=3  IndexOptions=Index vector (dialog)  Indices=[3 2 1]  OutputSizes=1
  Terminator : Terminator
  Transfer Fcn : TransferFcn  Denominator=[.01 1]
  Transfer Fcn1 : TransferFcn  Denominator=[.01 1]
  Transpose : Math  Operator=transpose  SignedPower=on
  Wind_e : Outport  Unit=m/s  VectorParamsAs1DForOutWhenUnconnected=off
  Rho : Outport  Port=2  VectorParamsAs1DForOutWhenUnconnected=off
  wires:
  Bus Selector/1 -> Transfer Fcn1/1  "<airspeed>"
  AirData/1 -> Bus Selector/1
  Transfer Fcn/1 -> Gain/1
  Dryden Wind Turbulence Model (Discrete (+q -r))/2 -> Terminator/1
  Reduce Z Wind/1 -> Add/1
  Dryden Wind Turbulence Model (Discrete (+q -r))/1 -> Reduce Z Wind/1
  Rotate to E Frame/1 -> Wind_e/1
  Transpose/1 -> Rotate to E Frame/1
  Horizontal Wind Model/1 -> Add/2
  Transfer Fcn1/1 -> Dryden Wind Turbulence Model (Discrete (+q -r))/2
  Add/1 -> Rotate to E Frame/2
  Rotation Angles to Direction Cosine Matrix/1 -> Dryden Wind Turbulence Model (Discrete (+q -r))/3, Horizontal Wind Model/1, Transpose/1  "RECEF2B"
  Get Z/1 -> Transfer Fcn/1
  Xe/1 -> Get Z/1
  Gain/1 -> Dryden Wind Turbulence Model (Discrete (+q -r))/1
  Constant1/1 -> Rho/1
  Selector/1 -> Rotation Angles to Direction Cosine Matrix/1
  Euler/1 -> Selector/1

== system VTOLDynamics/Force and Moments/Aerodynamic Forces/Compute Body Frame Forces and Moments/Wind frame F& M ==
  Airdata : Inport
  CtrlSurfaces : Inport  Port=2
  p,q,r : Inport  Port=3
  Bus Selector : BusSelector  OutputSignals=q
  Bus Selector1 : BusSelector  OutputSignals=dA,dR
  Bus Selector2 : BusSelector  OutputSignals=dE,dA,dR
  Bus Selector6 : BusSelector  OutputSignals=beta,airspeed
  Bus Selector7 : BusSelector  OutputSignals=alpha,airspeed
  Lateral Channel : Subsystem
  Longitudinal Channel : Subsystem
  Mux : Mux  Inputs=6
  Route coefficients : Subsystem
  coef : Outport  PortDimensions=6  VectorParamsAs1DForOutWhenUnconnected=off
  q : Outport  Port=2
  wires:
  Bus Selector7/2 -> Longitudinal Channel/2(Airpseed)  "<airspeed>"
  Bus Selector7/1 -> Longitudinal Channel/1(alpha)  "<alpha>"
  Bus Selector6/2 -> Lateral Channel/2(Airspeed)  "<airspeed>"
  Bus Selector6/1 -> Lateral Channel/1(beta)  "<beta>"
  Airdata/1 -> Bus Selector/1, Bus Selector6/1, Bus Selector7/1
  Bus Selector2/1 -> Longitudinal Channel/3(dE)  "<dE>"
  Bus Selector1/2 -> Lateral Channel/4(dR)  "<dR>"
  Bus Selector1/1 -> Lateral Channel/3(dA)  "<dA>"
  CtrlSurfaces/1 -> Bus Selector1/1, Bus Selector2/1
  p,q,r/1 -> Lateral Channel/5(p,q,r), Longitudinal Channel/4(p,q,r)
  Bus Selector2/2 -> Longitudinal Channel/5(dA)  "<dA>"
  Bus Selector2/3 -> Longitudinal Channel/6(dR)  "<dR>"
  Mux/1 -> coef/1
  Lateral Channel/1(Lateral) -> Route coefficients/1(Lateral)
  Longitudinal Channel/1(Longitudinal) -> Route coefficients/2(Longitudinal)
  Route coefficients/1(<CD>) -> Mux/1
  Route coefficients/2(<CY>) -> Mux/2
  Route coefficients/3(<CL>) -> Mux/3
  Route coefficients/4(<Cl>) -> Mux/4
  Route coefficients/5(<Cm>) -> Mux/5
  Route coefficients/6(<Cn>) -> Mux/6
  Bus Selector/1 -> q/1  "<q>"

== system VTOLDynamics/Force and Moments/Ground Model/Friction Force/Soft Coulomb Friction ==
  note: Pennestrì, E., Rossi, V., Salvini, P. et al. Review and comparison of dry friction force models. Nonlinear Dyn 83, 1785–1801 (2016). https://doi.org/10.1007/s11071-015-2485-3
  V : Inport
  Tanh : Trigonometry  Operator=tanh
  friction coefficient : Gain  Gain=contact.rollingFriction*1.2
  vd : Gain  Gain=1/contact.vd
  Out1 : Outport
  wires:
  V/1 -> vd/1
  vd/1 -> Tanh/1
  Tanh/1 -> friction coefficient/1
  friction coefficient/1 -> Out1/1

== system VTOLDynamics/Force and Moments/Propulsion/Electric Propulsion/Energy ==
  note: Range Estimator
  s : Inport
  Add : Sum  Inputs=++++
  Add1 : Sum
  Bus Selector : BusSelector  OutputSignals=Info1,Info2,Info3,Info4,airspeed,Current,Volt
  Constant3 : Constant  Value=0.01
  Display : Display
  Display1 : Display
  Distance : Subsystem
  Energy Motor1 : Subsystem
  Energy Motor2 : Subsystem
  Energy Motor3 : Subsystem
  Energy Motor4 : Subsystem
  Online Range : Subsystem
  Range Rating : Subsystem
  Terminator : Terminator
  wires:
  Bus Selector/1 -> Energy Motor1/1(M1)  "<Info1>"
  Bus Selector/2 -> Energy Motor2/1(M2)  "<Info2>"
  Bus Selector/3 -> Energy Motor3/1(M3)  "<Info3>"
  Bus Selector/4 -> Energy Motor4/1(M4)  "<Info4>"
  Energy Motor2/1(E2) -> Add/2
  Energy Motor3/1(E3) -> Add/3
  Energy Motor4/1(E4) -> Add/4
  Add/1 -> Display1/1
  Energy Motor1/1(E1) -> Add/1
  Distance/1(Dist) -> Add1/2
  Add1/1 -> Range Rating/1(d)
  Distance/2(SimTime(s)) -> Terminator/1
  Constant3/1 -> Add1/1
  Online Range/1(E) -> Range Rating/2(E), Display/1
  s/1 -> Bus Selector/1
  Bus Selector/5 -> Distance/1(VehSpd)  "<airspeed>"
  Bus Selector/7 -> Online Range/2(V)  "<Volt>"
  Bus Selector/6 -> Online Range/1(I)  "<Current>"

== system VTOLDynamics/Force and Moments/Propulsion/Electric Propulsion/Tilt Servo Dynamics ==
  TiltA : Inport
  TiltB : Inport  Port=2
  Gain2 : Gain  Gain=pi/2
  Gain3 : Gain  Gain=pi/2
  IC : InitialCondition  Value=tiltIni
  IC1 : InitialCondition  Value=tiltIni
  Servo Dynamics : TransferFcn  Denominator=[0.1 1]
  Servo Dynamics1 : TransferFcn  Denominator=[0.1 1]
  Tilt1 : Outport
  Tilt2 : Outport  Port=2
  wires:
  TiltA/1 -> Gain2/1
  Gain3/1 -> Servo Dynamics1/1
  IC1/1 -> Tilt1/1  "Tilt1"
  IC/1 -> Tilt2/1  "Tilt2"
  Servo Dynamics1/1 -> IC/1
  Servo Dynamics/1 -> IC1/1
  TiltB/1 -> Gain3/1
  Gain2/1 -> Servo Dynamics/1

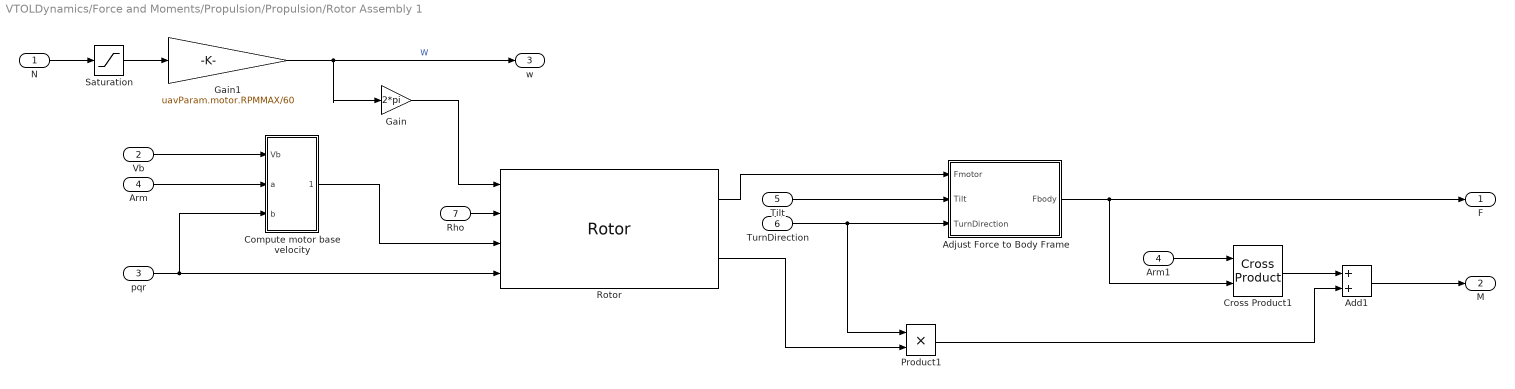
== system VTOLDynamics/Force and Moments/Propulsion/Propulsion/Rotor Assembly 1 ==
  N : Inport
  Vb : Inport  Port=2
  pqr : Inport  Port=3
  Arm : Inport  Port=4
  Tilt : Inport  Port=5
  TurnDirection : Inport  Port=6
  Rho : Inport  Port=7
  Add1 : Sum
  Adjust Force to Body Frame : Subsystem
  Arm1 : InportShadow  Port=4
  Compute motor base velocity : Subsystem
  Cross Product1 : matrix_library/Cross Product
  Gain : Gain  Gain=2*pi
  Gain1 : Gain  Gain=uavParam.motor.RPMMAX/60
  Product1 : Product
  Rotor : Rotor  modelMode=With flap effects  CT=4/(pi^3)*0.1142  CQ=8/(pi^3)*0.007048  radius=uavParam.geom.PropDiameter/2
      settings: LibrarySourceBlock=aerolibrotor/Rotor
  Saturation : Saturate  UpperLimit=1  LowerLimit=minPWM
  F : Outport
  M : Outport  Port=2
  w : Outport  Port=3
  wires:
  TurnDirection/1 -> Adjust Force to Body Frame/3(TurnDirection), Product1/1
  Adjust Force to Body Frame/1(Fbody) -> Cross Product1/2, F/1
  Compute motor base velocity/1(Vmotor) -> Rotor/3
  Arm/1 -> Compute motor base velocity/2(a)
  Vb/1 -> Compute motor base velocity/1(Vb)
  Product1/1 -> Add1/2
  Cross Product1/1 -> Add1/1
  Arm1/1 -> Cross Product1/1
  Rho/1 -> Rotor/2
  Add1/1 -> M/1
  Rotor/2 -> Product1/2
  Gain/1 -> Rotor/1
  pqr/1 -> Rotor/4, Compute motor base velocity/3(b)
  Saturation/1 -> Gain1/1
  N/1 -> Saturation/1
  Gain1/1 -> w/1, Gain/1  "W"
  Tilt/1 -> Adjust Force to Body Frame/2(Tilt)
  Rotor/1 -> Adjust Force to Body Frame/1(Fmotor)

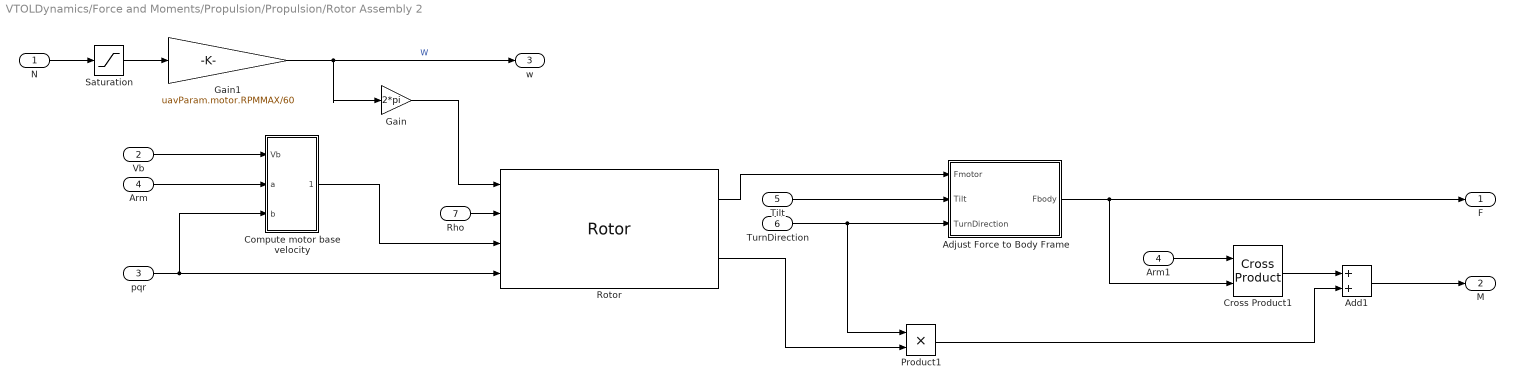
== system VTOLDynamics/Force and Moments/Propulsion/Propulsion/Rotor Assembly 2 ==
  N : Inport
  Vb : Inport  Port=2
  pqr : Inport  Port=3
  Arm : Inport  Port=4
  Tilt : Inport  Port=5
  TurnDirection : Inport  Port=6
  Rho : Inport  Port=7
  Add1 : Sum
  Adjust Force to Body Frame : Subsystem
  Arm1 : InportShadow  Port=4
  Compute motor base velocity : Subsystem
  Cross Product1 : matrix_library/Cross Product
  Gain : Gain  Gain=2*pi
  Gain1 : Gain  Gain=uavParam.motor.RPMMAX/60
  Product1 : Product
  Rotor : Rotor  modelMode=With flap effects  CT=4/(pi^3)*0.1142  CQ=8/(pi^3)*0.007048  radius=uavParam.geom.PropDiameter/2
      settings: LibrarySourceBlock=aerolibrotor/Rotor
  Saturation : Saturate  UpperLimit=1  LowerLimit=minPWM
  F : Outport
  M : Outport  Port=2
  w : Outport  Port=3
  wires:
  Gain1/1 -> Gain/1, w/1  "W"
  N/1 -> Saturation/1
  Saturation/1 -> Gain1/1
  pqr/1 -> Rotor/4, Compute motor base velocity/3(b)
  Gain/1 -> Rotor/1
  Rotor/2 -> Product1/2
  Add1/1 -> M/1
  Rho/1 -> Rotor/2
  Arm1/1 -> Cross Product1/1
  Cross Product1/1 -> Add1/1
  Product1/1 -> Add1/2
  Vb/1 -> Compute motor base velocity/1(Vb)
  Arm/1 -> Compute motor base velocity/2(a)
  Compute motor base velocity/1(Vmotor) -> Rotor/3
  Adjust Force to Body Frame/1(Fbody) -> F/1, Cross Product1/2
  TurnDirection/1 -> Product1/1, Adjust Force to Body Frame/3(TurnDirection)
  Tilt/1 -> Adjust Force to Body Frame/2(Tilt)
  Rotor/1 -> Adjust Force to Body Frame/1(Fmotor)

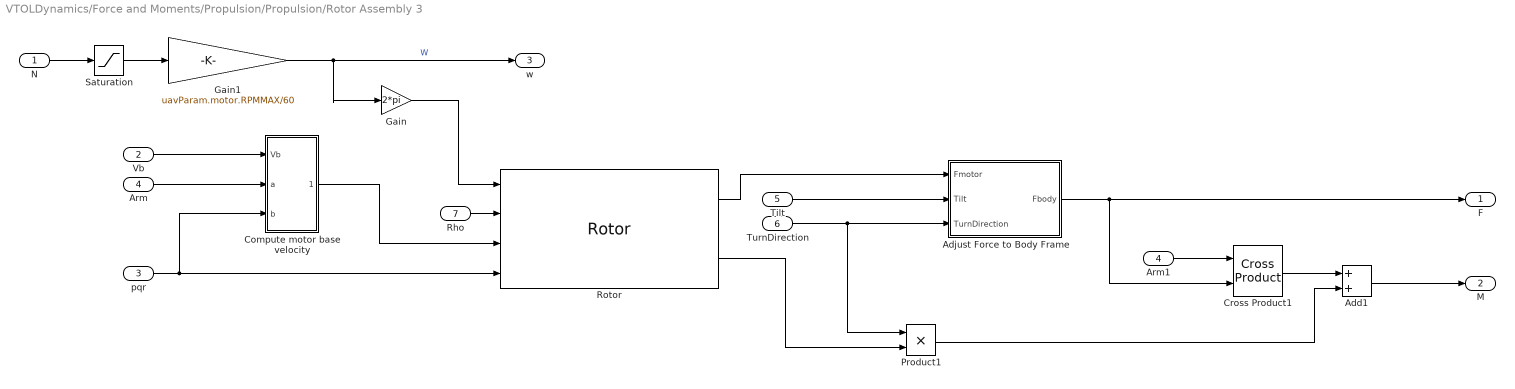
== system VTOLDynamics/Force and Moments/Propulsion/Propulsion/Rotor Assembly 3  ==
  N : Inport
  Vb : Inport  Port=2
  pqr : Inport  Port=3
  Arm : Inport  Port=4
  Tilt : Inport  Port=5
  TurnDirection : Inport  Port=6
  Rho : Inport  Port=7
  Add1 : Sum
  Adjust Force to Body Frame : Subsystem
  Arm1 : InportShadow  Port=4
  Compute motor base velocity : Subsystem
  Cross Product1 : matrix_library/Cross Product
  Gain : Gain  Gain=2*pi
  Gain1 : Gain  Gain=uavParam.motor.RPMMAX/60
  Product1 : Product
  Rotor : Rotor  modelMode=With flap effects  CT=4/(pi^3)*0.1142  CQ=8/(pi^3)*0.007048  radius=uavParam.geom.PropDiameter/2
      settings: LibrarySourceBlock=aerolibrotor/Rotor
  Saturation : Saturate  UpperLimit=1  LowerLimit=minPWM
  F : Outport
  M : Outport  Port=2
  w : Outport  Port=3
  wires:
  TurnDirection/1 -> Adjust Force to Body Frame/3(TurnDirection), Product1/1
  Adjust Force to Body Frame/1(Fbody) -> Cross Product1/2, F/1
  Compute motor base velocity/1(Vmotor) -> Rotor/3
  Arm/1 -> Compute motor base velocity/2(a)
  Vb/1 -> Compute motor base velocity/1(Vb)
  Product1/1 -> Add1/2
  Cross Product1/1 -> Add1/1
  Arm1/1 -> Cross Product1/1
  Rho/1 -> Rotor/2
  Add1/1 -> M/1
  Rotor/2 -> Product1/2
  Gain/1 -> Rotor/1
  pqr/1 -> Rotor/4, Compute motor base velocity/3(b)
  Saturation/1 -> Gain1/1
  N/1 -> Saturation/1
  Gain1/1 -> w/1, Gain/1  "W"
  Tilt/1 -> Adjust Force to Body Frame/2(Tilt)
  Rotor/1 -> Adjust Force to Body Frame/1(Fmotor)

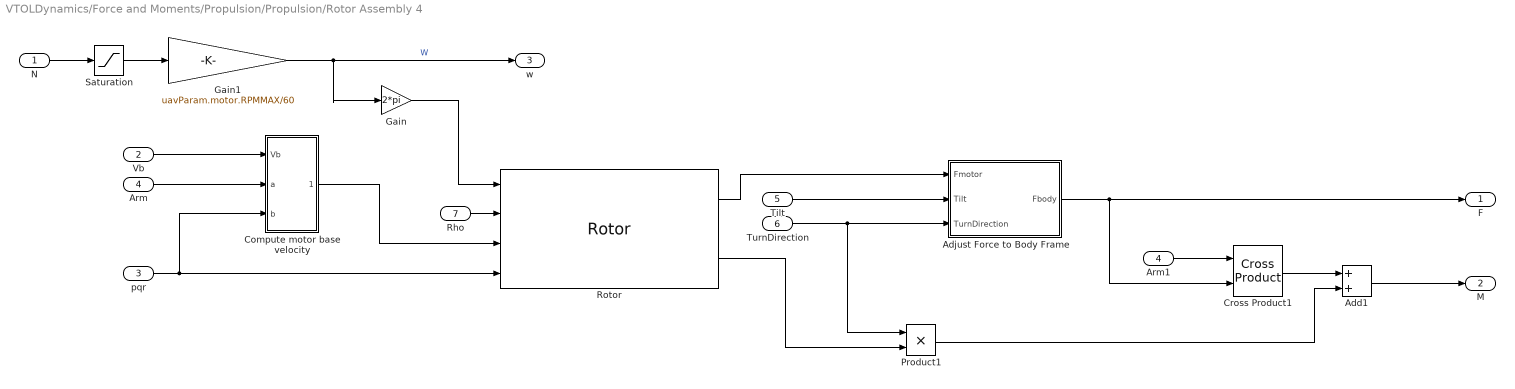
== system VTOLDynamics/Force and Moments/Propulsion/Propulsion/Rotor Assembly 4 ==
  N : Inport
  Vb : Inport  Port=2
  pqr : Inport  Port=3
  Arm : Inport  Port=4
  Tilt : Inport  Port=5
  TurnDirection : Inport  Port=6
  Rho : Inport  Port=7
  Add1 : Sum
  Adjust Force to Body Frame : Subsystem
  Arm1 : InportShadow  Port=4
  Compute motor base velocity : Subsystem
  Cross Product1 : matrix_library/Cross Product
  Gain : Gain  Gain=2*pi
  Gain1 : Gain  Gain=uavParam.motor.RPMMAX/60
  Product1 : Product
  Rotor : Rotor  modelMode=With flap effects  CT=4/(pi^3)*0.1142  CQ=8/(pi^3)*0.007048  radius=uavParam.geom.PropDiameter/2
      settings: LibrarySourceBlock=aerolibrotor/Rotor
  Saturation : Saturate  UpperLimit=1  LowerLimit=minPWM
  F : Outport
  M : Outport  Port=2
  w : Outport  Port=3
  wires:
  Gain1/1 -> Gain/1, w/1  "W"
  N/1 -> Saturation/1
  Saturation/1 -> Gain1/1
  pqr/1 -> Rotor/4, Compute motor base velocity/3(b)
  Gain/1 -> Rotor/1
  Rotor/2 -> Product1/2
  Add1/1 -> M/1
  Rho/1 -> Rotor/2
  Arm1/1 -> Cross Product1/1
  Cross Product1/1 -> Add1/1
  Product1/1 -> Add1/2
  Vb/1 -> Compute motor base velocity/1(Vb)
  Arm/1 -> Compute motor base velocity/2(a)
  Compute motor base velocity/1(Vmotor) -> Rotor/3
  Adjust Force to Body Frame/1(Fbody) -> F/1, Cross Product1/2
  Rotor/1 -> Adjust Force to Body Frame/1(Fmotor)
  TurnDirection/1 -> Product1/1, Adjust Force to Body Frame/3(TurnDirection)
  Tilt/1 -> Adjust Force to Body Frame/2(Tilt)

== system VTOLDynamics/Force and Moments/Propulsion/Propulsion/Tilt Servo Dynamics ==
  TiltA : Inport
  TiltB : Inport  Port=2
  Gain2 : Gain  Gain=pi/2
  Gain3 : Gain  Gain=pi/2
  IC : InitialCondition  Value=tiltIni
  IC1 : InitialCondition  Value=tiltIni
  Servo Dynamics : TransferFcn  Denominator=[0.1 1]
  Servo Dynamics1 : TransferFcn  Denominator=[0.1 1]
  Tilt1 : Outport
  Tilt2 : Outport  Port=2
  wires:
  Gain2/1 -> Servo Dynamics/1
  TiltB/1 -> Gain3/1
  Servo Dynamics/1 -> IC1/1
  Servo Dynamics1/1 -> IC/1
  IC/1 -> Tilt2/1  "Tilt2"
  IC1/1 -> Tilt1/1  "Tilt1"
  Gain3/1 -> Servo Dynamics1/1
  TiltA/1 -> Gain2/1

== system VTOLDynamics/Force and Moments/Aerodynamic Forces/Compute Body Frame Forces and Moments/Wind frame F& M/Lateral Channel ==
  beta : Inport
  Airspeed : Inport  Port=2
  dA : Inport  Port=3
  dR : Inport  Port=4
  p,q,r : Inport  Port=5
  Bus Creator : BusCreator  Inputs=3
  CY : Subsystem
  Cl : Subsystem
  Cn : Subsystem
  Lateral : Outport  VectorParamsAs1DForOutWhenUnconnected=off
  wires:
  Cl/1(Cl) -> Bus Creator/2  "Cl"
  p,q,r/1 -> CY/3(p,q,r), Cn/4(p,q,r), Cl/4(p,q,r)
  Airspeed/1 -> CY/4(Airspeed), Cn/5(Airspeed), Cl/5(Airspeed)
  dR/1 -> CY/2(dR), Cl/3(dR), Cn/3(dR)
  dA/1 -> Cl/2(dA), Cn/2(dA)
  beta/1 -> CY/1(beta), Cl/1(beta), Cn/1(beta)
  Cn/1(Cn) -> Bus Creator/3  "Cn"
  CY/1(CY) -> Bus Creator/1  "CY"
  Bus Creator/1 -> Lateral/1

== system VTOLDynamics/Force and Moments/Aerodynamic Forces/Compute Body Frame Forces and Moments/Wind frame F& M/Longitudinal Channel ==
  alpha : Inport
  Airpseed : Inport  Port=2
  dE : Inport  Port=3
  p,q,r : Inport  Port=4
  dA : Inport  Port=5
  dR : Inport  Port=6
  Bus Creator : BusCreator  Inputs=3
  CD : Subsystem
  CL : Subsystem
  Cm : Subsystem
  Saturation : Saturate  UpperLimit=14*pi/180  LowerLimit=-14*pi/180  LinearizeAsGain=off  ZeroCross=off
  Transfer Fcn : TransferFcn  Numerator=[1 0]  Denominator=[0.1 1]
  Y-down : Gain  SaturateOnIntegerOverflow=on  OutDataTypeStr=Inherit: Same as input  ParamDataTypeStr=Inherit: Same as input
      settings: AttributesFormatString=%<Gain>
  Longitudinal : Outport  VectorParamsAs1DForOutWhenUnconnected=off
  wires:
  Transfer Fcn/1 -> CL/2(alpha_dot)
  Airpseed/1 -> Cm/4(Airspeed), CL/5(Airspeed)
  p,q,r/1 -> Cm/3(p,q,r), CL/4(p,q,r)
  Bus Creator/1 -> Longitudinal/1
  Cm/1(Cm) -> Bus Creator/3  "Cm"
  CL/1(CL) -> CD/1(CL), Y-down/1
  dE/1 -> Cm/2(De), CD/4(dE), CL/3(dE)
  Y-down/1 -> Bus Creator/2  "CL"
  CD/1(CD) -> Bus Creator/1  "CD"
  alpha/1 -> Saturation/1
  dR/1 -> CD/3(dR)
  dA/1 -> CD/2(dA), CL/6(dA)
  Saturation/1 -> Transfer Fcn/1, Cm/1(alpha), CL/1(alpha)

== system VTOLDynamics/Force and Moments/Aerodynamic Forces/Compute Body Frame Forces and Moments/Wind frame F& M/Route coefficients ==
  Lateral : Inport
  Longitudinal : Inport  Port=2
  Bus Selector : BusSelector  OutputSignals=CY,Cl,Cn
  Bus Selector3 : BusSelector  OutputSignals=CD,CL,Cm
  <CD> : Outport
  <CY> : Outport  Port=2
  <CL> : Outport  Port=3
  <Cl> : Outport  Port=4
  <Cm> : Outport  Port=5
  <Cn> : Outport  Port=6
  wires:
  Bus Selector3/2 -> <CL>/1  "<CL>"
  Bus Selector/3 -> <Cn>/1  "<Cn>"
  Bus Selector/2 -> <Cl>/1  "<Cl>"
  Lateral/1 -> Bus Selector/1
  Bus Selector3/3 -> <Cm>/1  "<Cm>"
  Bus Selector3/1 -> <CD>/1  "<CD>"
  Longitudinal/1 -> Bus Selector3/1
  Bus Selector/1 -> <CY>/1  "<CY>"

== system VTOLDynamics/Force and Moments/Propulsion/Electric Propulsion/Energy/Distance ==
  VehSpd : Inport
  Add : Sum
  Constant : Constant
  Constant1 : Constant  Value=0.1
  Display : Display
  Divide : Product  Inputs=*/
  Integrator : Integrator
  Integrator1 : Integrator
  Dist : Outport
  SimTime(s) : Outport  Port=2
  wires:
  Divide/1 -> Display/1
  Integrator/1 -> Dist/1, Divide/1  "Distance"
  VehSpd/1 -> Integrator/1
  Add/1 -> SimTime(s)/1, Divide/2
  Integrator1/1 -> Add/1  "time"
  Constant1/1 -> Add/2
  Constant/1 -> Integrator1/1

== system VTOLDynamics/Force and Moments/Propulsion/Electric Propulsion/Energy/Energy Motor1 ==
  Bus Element In : Inport  PortName=M1  Element=Current
  Bus Element In1 : Inport  PortName=M1  Element=Volt
  Integrator : Integrator
  Product : Product
  E1 : Outport
  wires:
  Bus Element In/1 -> Product/1
  Bus Element In1/1 -> Product/2
  Product/1 -> Integrator/1
  Integrator/1 -> E1/1

== system VTOLDynamics/Force and Moments/Propulsion/Electric Propulsion/Energy/Energy Motor2 ==
  Bus Element In : Inport  PortName=M2  Element=Current
  Bus Element In1 : Inport  PortName=M2  Element=Volt
  Integrator : Integrator
  Product : Product
  E2 : Outport
  wires:
  Integrator/1 -> E2/1
  Product/1 -> Integrator/1
  Bus Element In1/1 -> Product/2
  Bus Element In/1 -> Product/1

== system VTOLDynamics/Force and Moments/Propulsion/Electric Propulsion/Energy/Energy Motor3 ==
  Bus Element In : Inport  PortName=M3  Element=Current
  Bus Element In1 : Inport  PortName=M3  Element=Volt
  Integrator : Integrator
  Product : Product
  E3 : Outport
  wires:
  Bus Element In/1 -> Product/1
  Bus Element In1/1 -> Product/2
  Product/1 -> Integrator/1
  Integrator/1 -> E3/1

== system VTOLDynamics/Force and Moments/Propulsion/Electric Propulsion/Energy/Energy Motor4 ==
  Bus Element In : Inport  PortName=M4  Element=Current
  Bus Element In1 : Inport  PortName=M4  Element=Volt
  Integrator : Integrator
  Product : Product
  E4 : Outport
  wires:
  Integrator/1 -> E4/1
  Product/1 -> Integrator/1
  Bus Element In1/1 -> Product/2
  Bus Element In/1 -> Product/1
